simulink model "lab8_model"  (R2022a)
settings: Solver=FixedStepAuto  StartTime=0.0  StopTime=150  FixedStep=0.001  RelTol=1e-3
values from neighbouring files (symbols this model uses):
  b1 = (gv1 * km) / A^2    [Lab8.m]    (also in linear_workspace.mat = 0.0153089919564; nonlinear_workspace.mat = 0.0153089919564)
  b2 = (gv1 + gv2) / A    [Lab8.m]    (also in linear_workspace.mat = 0.132188122222; nonlinear_workspace.mat = 0.132188122222)
  b3 = (gv1 *gv2) / A^2    [Lab8.m]    (also in linear_workspace.mat = 0.00436679419784; nonlinear_workspace.mat = 0.00436679419784)
  Kd = (2*zeta*omega + alpha - b2) / b1    [Lab8.m]    (also in linear_workspace.mat = 34.2521231491; nonlinear_workspace.mat = 34.2521231491)
  Ki = (alpha*omega^2) / b1    [Lab8.m]    (also in linear_workspace.mat = 0.514641540244; nonlinear_workspace.mat = 0.514641540244)
  Kp = (omega^2 + 2*alpha*zeta*omega - b3) / b1    [Lab8.m]    (also in linear_workspace.mat = 4.56614097638; nonlinear_workspace.mat = 4.56614097638)
settings Model: Creator=ahmcmillon  LastModifiedBy=ahmcmillon
settings DataIOCC: ReturnWorkspaceOutputs=off

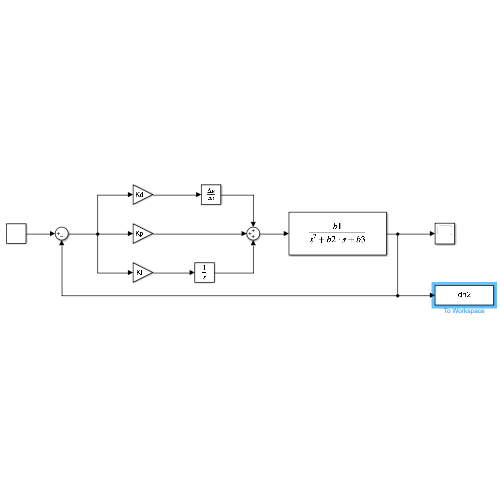
[thumbnail: Simulink's stored preview of the top-level diagram]
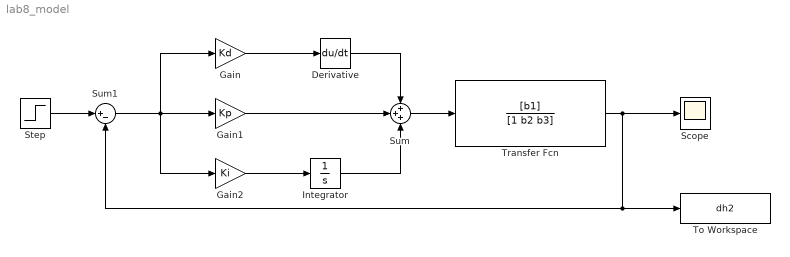
== system lab8_model ==
  Derivative : Derivative
  Gain : Gain  Gain=Kd
  Gain1 : Gain  Gain=Kp
  Gain2 : Gain  Gain=Ki
  Integrator : Integrator
  Scope : Scope
  Step : Step  Time=0  After=2  SampleTime=0
  Sum : Sum  Inputs=+++
  Sum1 : Sum  Inputs=|+-
  To Workspace : ToWorkspace  VariableName=dh2  SaveFormat=Structure With Time  SampleTime=-1
  Transfer Fcn : TransferFcn  Numerator=[b1]  Denominator=[1 b2 b3]
  wires:
  Step/1 -> Sum1/1
  Sum1/1 -> Gain2/1, Gain/1, Gain1/1
  Gain2/1 -> Integrator/1
  Gain1/1 -> Sum/2
  Integrator/1 -> Sum/3
  Gain/1 -> Derivative/1
  Derivative/1 -> Sum/1
  Sum/1 -> Transfer Fcn/1
  Transfer Fcn/1 -> Sum1/2, To Workspace/1, Scope/1
